simulink model "BiT_Template"  (R2025b)
settings: Solver=FixedStepAuto  StartTime=0.0  StopTime=40  FixedStep=0.005  RelTol=1e-3
StopFcn:
  | user_confirmed = true;
  | disp('Gestoppt?!')
  | 
  | % stop(t);
  | % delete(t);
  | 
  | %% Switch to Config Mode
  | %Tc3_AI.sysManager.ActivateConfiguration();
  | %
  | % Tc3_AI.SwitchToConfig('local')
  | %
  | % %save Solution
  | % Tc3_AI.SaveSolution();
  | %
  | % %% Close Aktive VS Instance
  | % Tc3_AI.closeVsInstance();
libraries: slpidlib x1
settings Model: SimulationMode=external  Creator=clemensm  LastModifiedBy=Felix
settings OptimizationCC: LocalBlockOutputs=off
settings RTWCC: SystemTargetFile=TwinCatGrt.tlc  GenCodeOnly=on  GenerateMakefile=off  TemplateMakefile=tcgrt_msbuild.tmf  TargetLang=C++  Description=TwinCAT GRT Target
settings STFCustomTargetCC: SystemTargetFile=TwinCatGrt.tlc  TargetLangStandard=C++11 (ISO)  CombineOutputUpdateFcns=on  CodeInterfacePackaging=Reusable function  CPPClassGenCompliant=on  GRTInterface=off  GenerateAllocFcn=on  TcCom_BlockDiagramExport=on  TcCom_Legacy_ModuleBuildInfoParam=on  TcCom_ExtModeRtWaitForStart=off  TcProject_LibraryCategories=$<VendorName>  TcCom_ExecutionSequence=UpdateBeforeOutputMapping  TcProject_UseTmxExtension=Auto  TcCom_OnlineChange=off  TcProject_ProjectDir=C:\TwinCAT\3.1\CustomConfig\Modules\Ctrl_only  TcCom_AllowDataAreaForSharedData=off  TcCom_TcComWrapperFb=off  TcProject_VendorIcon=$<TE140x:Icon>  TcProject_Copyright=Copyright $<VendorName> $<LocalDateTime:%Y>  TcProject_UseNativeBlockDiagramExport=off  TcProject_LowestCompatibleTcBuild=$<TwinCAT:Version:BUILD>  TcCom_BlockIoDataAccess=Internal DataArea  TcCom_ModuleIcon=$<TE140x:Icon>  TcPlcFb_ExtModeRtWaitForStart=off  TcPlcFb_ExtModeRtAllowExecutionCommands=off  TcCom_DataStoreReadOnly=off  TcProject_GenerateStructDutsWithDefaultValues=Auto  TcProject_InstallPlcLibrary=off  TcPlcFb_ExtModeRtAllowForParameterChange=off  TcPlcFb_InitExceptionHandling=CallerExceptions  TcCom_ExecutionInfoParam=on  TcCom_DWorkReadOnly=on  TcCom_CallerVerification=Default  TcProject_BuildWithWdk=inherit default  TcCom_BlockDiagramVariableAccess=AssignToParent  TcCom_TcComWrapperFbProperties=off  TcProject_UseIntrinsics=on  TcCom_InputCreateSymbols=on  TcProject_ForceRebuildForPublish=off  TcProject_CLanguageStandard=Default  TcCom_DWorkCreateSymbols=on  TcCom_OemLicenses=$<Project:OemLicenses>  TcCom_ExtendSignalResolution=on  TcProject_PublishTcOSARMv7M=off  TcProject_PreferToolArchitectureX64=on  TcCom_StepSizeAdaptation=RequireMatchingTaskCycleTime  TcPlcFb_Generate=off  TcCom_OnlineChangeRestoreDataAreas=off  TcProject_PreferIntOverLong=off  TcProject_CoderCppNamespace=coder  TcProject_Generate=on  TcCom_OutputReadOnly=on  TcProject_CreateUniqueEnumItemNames=off  TcCom_DataStoreCreateSymbols=on  TcProject_UseDescriptorCodeType=on  TcCom_TcComWrapperFbPropertyMonitoring=NoMonitoring  TcProject_UseStaticStlString=off  TcProject_Description=TwinCAT executable file, generated by TwinCAT $<ModuleGenerator:ProductId>  TcPlcFb_MonitorExecutionTime=off  TcCom_DWorkDataAccess=Internal DataArea  TcCom_InputInitValues=off  TcProject_UseCodeDescriptor=on  TcCom_GlobalParamDefaultSharing=Define  TcCom_BlockDiagramDebugInfoExport=on  TcProject_SignTwinCatCertName=MCI_2024_OEM.tccert  TcProject_StaticStlStringCapacity=Auto  TcCom_ContStateReadOnly=on  TcCom_UpdateExceptionHandling=CallerExceptions  TcProject_DrvFileVersion=$<VersionFromFile>  TcCom_ExtModeRtAllowForParameterChange=on  TcCom_VariableSymbolMapping=Identical  TcCom_BlockIoReadOnly=on  TcCom_ExecuteModelCode=on  TcCom_OutputDataAccess=Output Source DataArea  TcCom_BlockIoCreateSymbols=on  TcProject_GeneratePlcLibrary=off  TcProject_PublishTcOSARMv8A=off  TcProject_PublishTcOSx64=off  TcProject_DeployRestart=off  TcProject_ClassFactoryName=$<Project:Name>  TcProject_PublishConfiguration=Release  TcProject_IncrementVersion=Revision  TcProject_Versioning=Versioned  TcProject_BuildSystem=Auto  TcCom_ExtModeRtAllowExecutionCommands=on  TcProject_LibCatPath=$<Project:Dir>\$<Project:Name>.libcat.xml  TcCom_ParametersDataAccess=Internal DataArea  TcCom_ModuleCaller=CyclicTask  TcProject_TmxInstall=on  TcProject_PublishParallel=on  TcCom_ParametersInitValues=on  TcCom_AccessLockState=Auto  TcCom_InitExceptionHandling=CallerExceptions  TcCom_GroupDisplayName=$<GroupName>  TcCom_Generate=on  TcProject_PublishTcRTx86=on  TcProject_ProductName=$<ModuleGenerator:ProductId> $<ModuleGenerator:Version:MAJOR.MINOR>  TcCom_ExecutionInfoOutput=off  TcCom_GroupName=TE140x|Simulink Modules  TcProject_VersionSrc=$<LatestTMFile>  TcCom_ParametersCreateSymbols=on  TcCom_InputReadOnly=off  TcProject_PlcVarPrefixes=PVOID=p | BOOL=b | BOOL32=b | DATE=d | TIME_OF_DATE=td | TIME=t | LTIME=t | GUID=n  TcProject_Verbosity=Normal  TcProject_UseCodeInfoExporter=on  TcPlcFb_OemLicenses=$<Project:OemLicenses>  TcPlcFb_UpdateExceptionHandling=CallerExceptions  TcCom_StrictAccessLock=on  TcProject_Publish=on  TcCom_OriginalIoBlockNames=off  TcCom_ContStateDataAccess=Internal DataArea  TcCom_ResolveMaskedSubsystems=on  TcProject_MaxVisibleArrayElements=200U  TcCom_OutputCreateSymbols=on  TcProject_GenerateVsSolution=No  TcCom_DataStoreDataAccess=None  TcProject_PublishTcOSARMv7A=off  TcProject_CreateScopedEnums=Auto  TcCom_ParametersReadOnly=off  TcProject_SignWithTwinCatCertificate=inherit default  TcProject_PublishTcRTx64=on  TcProject_PublishPlatformtoolset=Auto  TcProject_EnableNewPlatforms=off  TcProject_DrvProductVersion=$<DrvFileVersion>  TcProject_PublishTcUMx86=off  TcProject_CppLanguageStandard=Default  TcCom_ContStateCreateSymbols=on  TcCom_InputDataAccess=Input Destination DataArea  TcCom_MonitorExecutionTime=off  TcProject_PublishTcUMx64=off  TcCom_GroupIcon=$<TE140x:Icon>  TcProject_DataExchangeModulesVersion=$<ModuleGenerator:DataExchange:Version>  TcProject_VendorName=TE140x Module Vendor  TcProject_UseDataExchangeModules=off
settings GRTTargetCC: ExtMode=on  ExtModeMexFile=TcExtModeClient  MultiInstanceErrorCode=None  TargetLangStandard=C++11 (ISO)  ParMdlRefBuildCompliant=off  CompOptLevelCompliant=off  MatFileLogging=off  CodeInterfacePackaging=Reusable function  GenerateAllocFcn=on  UseToolchainInfoCompliant=off

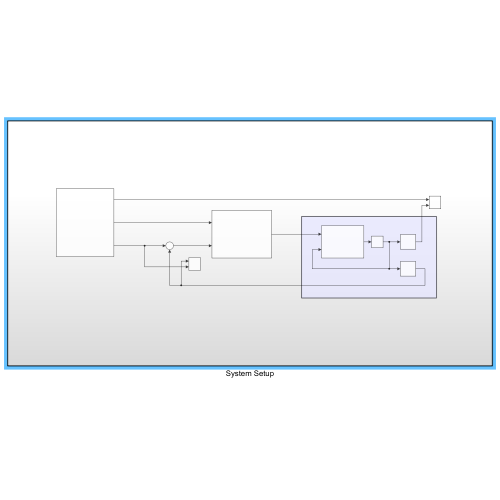
[thumbnail: Simulink's stored preview of the top-level diagram]
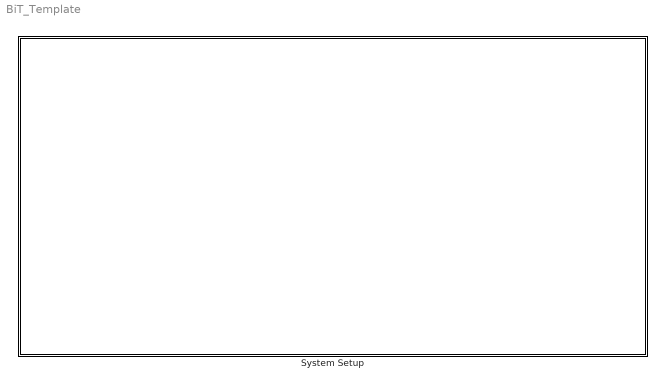
== system BiT_Template ==
  System Setup : Subsystem

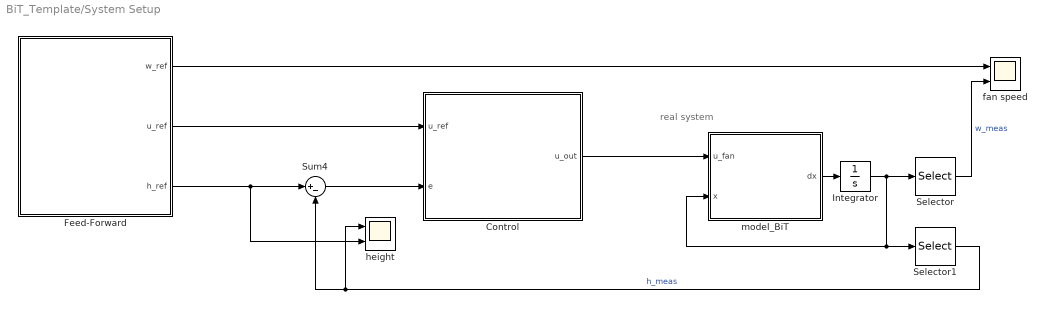
== system BiT_Template/System Setup ==
  note: real system
  Control : Subsystem
  Feed-Forward : Subsystem
  Integrator : Integrator
  Selector : Selector  InputPortWidth=3  IndexOptions=Index vector (dialog)  Indices=3  OutputSizes=1
  Selector1 : Selector  InputPortWidth=3  IndexOptions=Index vector (dialog)  Indices=1  OutputSizes=1
  Sum4 : Sum  Inputs=|+-
  fan speed : Scope  NumInputPorts=2
      settings: TimeSpan=60  ActiveDisplayYMinimum=4277  ActiveDisplayYMaximum=4777
  height : Scope  NumInputPorts=2
      settings: TimeSpan=60  ActiveDisplayYMinimum=-11.896668737884474  ActiveDisplayYMaximum=60.683450511895956  DataLoggingVariableName=ScopeData2
  model_BiT : MATLAB Function  TreatAsAtomicUnit=on
  wires:
  Selector1/1 -> height/1, Sum4/2  "h_meas"
  Selector/1 -> fan speed/2  "w_meas"
  model_BiT/1(dx) -> Integrator/1
  Integrator/1 -> Selector/1, Selector1/1, model_BiT/2(x)
  Feed-Forward/3(h_ref) -> height/2, Sum4/1
  Feed-Forward/1(w_ref) -> fan speed/1
  Feed-Forward/2(u_ref) -> Control/1(u_ref)
  Sum4/1 -> Control/2(e)
  Control/1(u_out) -> model_BiT/1(u_fan)

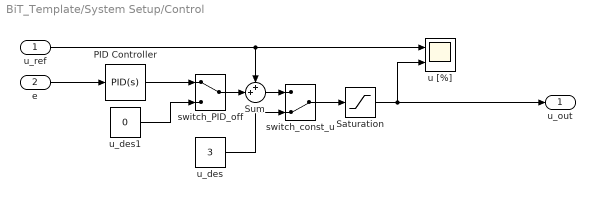
== system BiT_Template/System Setup/Control ==
  u_ref : Inport
  e : Inport  Port=2
  PID Controller : slpidlib/PID Controller  Controller=PID  Form=Parallel  TimeDomain=Continuous-time  UseExternalTs=off  SampleTime=-1  IntegratorMethod=Forward Euler  FilterMethod=Forward Euler  ControllerParametersSource=internal  P=1  I=1  UseKiTs=off  D=0  UseExternalDerivativeSource=off  N=100  UseFilter=on  TunerSelectOption=Transfer Function Based (PID Tuner App)  InitialConditionSource=internal  InitialConditionForIntegrator=0  InitialConditionForFilter=0  DifferentiatorICPrevScaledInput=0  ExternalReset=none  TrackingMode=off  Kt=1  LimitOutput=off  SatLimitsSource=internal  UpperSaturationLimit=inf  LowerSaturationLimit=-inf  LinearizeAsGain=on  AntiWindupMode=none  Kb=1  LimitIntegrator=off  UpperIntegratorSaturationLimit=inf  LowerIntegratorSaturationLimit=-inf  POutMin=[]  POutMax=[]  IOutMin=[]  IOutMax=[]  DOutMin=[]  DOutMax=[]  NOutMin=[]  NOutMax=[]  SumOutMin=[]  SumOutMax=[]  SaturationOutMin=[]  SaturationOutMax=[]  PParamMin=[]  PParamMax=[]  IParamMin=[]  IParamMax=[]  DParamMin=[]  DParamMax=[]  NParamMin=[]  NParamMax=[]  KbParamMin=[]  KbParamMax=[]  KtParamMin=[]  KtParamMax=[]  KbOutMin=[]  KbOutMax=[]  KtOutMin=[]  KtOutMax=[]  IntegratorOutMin=[]  IntegratorOutMax=[]  FilterOutMin=[]  FilterOutMax=[]  SumI1OutMin=[]  SumI1OutMax=[]  SumI2OutMin=[]  SumI2OutMax=[]  SumI3OutMin=[]  SumI3OutMax=[]  SumI4OutMin=[]  SumI4OutMax=[]  SumDOutMin=[]  SumDOutMax=[]  DifferentiatorOutMin=[]  DifferentiatorOutMax=[]  FilterDiffOutCoefMin=[]  FilterDiffOutCoefMax=[]  ReciprocalOutMin=[]  ReciprocalOutMax=[]  SumDenOutMin=[]  SumDenOutMax=[]  SumNumOutMin=[]  SumNumOutMax=[]  DivideOutMin=[]  DivideOutMax=[]  UdiffTsProdOutMin=[]  UdiffTsProdOutMax=[]  NTsProdOutMin=[]  NTsProdOutMax=[]  UintegralTsProdOutMin=[]  UintegralTsProdOutMax=[]  UngainTsProdOutMin=[]  UngainTsProdOutMax=[]  ClampingZeroOutDataTypeStr=Inherit: Inherit via back propagation  ClampingZeroOutMin=[]  ClampingZeroOutMax=[]  FilterDenConstantOutDataTypeStr=Inherit: Inherit via back propagation  FilterDenConstantOutMin=[]  FilterDenConstantOutMax=[]  PCopyOutDataTypeStr=Inherit: Inherit via back propagation  PCopyOutMin=[]  PCopyOutMax=[]  NCopyOutDataTypeStr=Inherit: Inherit via back propagation  NCopyOutMin=[]  NCopyOutMax=[]  IntegratorContinuousStateAttributes=''  IntegratorStateMustResolveToSignalObject=off  IntegratorRTWStateStorageClass=Auto  FilterContinuousStateAttributes=''  FilterStateMustResolveToSignalObject=off  FilterRTWStateStorageClass=Auto  ParallelPVariant=InternalParameters  IdealPVariant=Disabled  IVariant=InternalParameters  DVariant=InternalParameters  IntegratorVariant=Continuous  SatVariant=Disabled  AWVariant=Passthrough  PCopyVariant=Disabled  TRVariant=Disabled  FdbkBlocksVariant=Forward  IdealPFdbkVariant=Disabled  SatFdbkVariant=Disabled  DerivativeFilterVariant=ContFilter  NVariant=InternalParameters  NCopyVariant=Disabled  FilterICVariant=InternalICsFilter  IntegratorICVariant=InternalICs  ExternalResetVariant=Disabled  TRSumVariant=Passthrough  SumFdbkVariant=Disabled  SumVariant=Sum_PID  TsampFilterVariant=InternalTs  TsampNgainVariant=Passthrough  TsampIntegralVariant=Disabled_SignalSpec  ExternalSaturationOutDataTypeStr=Inherit: Same as second input  DerivativeSourceVariant=ErrorSignal  PreIntVariant=InternalPreInt
  Saturation : Saturate  UpperLimit=10  LowerLimit=0
  Sum : Sum  Inputs=++|
  switch_PID_off : ManualSwitch
  switch_const_u : ManualSwitch  CurrentSetting=0
  u [%] : Scope  NumInputPorts=2
      settings: TimeSpan=60  ActiveDisplayYMinimum=1.6341767510650569  ActiveDisplayYMaximum=6.6167058635554366
  u_des : Constant  Value=3
  u_des1 : Constant  Value=0
  u_out : Outport
  wires:
  u_des/1 -> switch_const_u/2
  Saturation/1 -> u_out/1, u [%]/2
  e/1 -> PID Controller/1
  switch_const_u/1 -> Saturation/1
  u_ref/1 -> u [%]/1, Sum/1
  Sum/1 -> switch_const_u/1
  PID Controller/1 -> switch_PID_off/1
  switch_PID_off/1 -> Sum/2
  u_des1/1 -> switch_PID_off/2

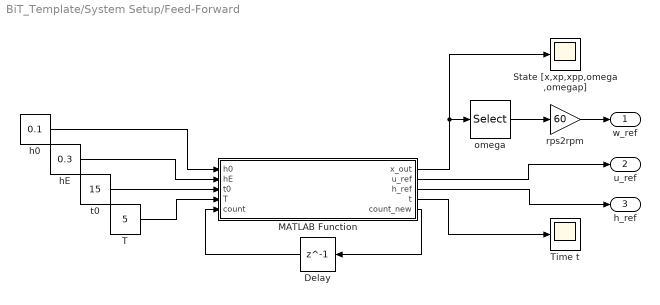
== system BiT_Template/System Setup/Feed-Forward ==
  Delay : Delay  DelayLength=1
  MATLAB Function : MATLAB Function  TreatAsAtomicUnit=on
  State [x,xp,xpp,omega,omegap] : Scope
      settings: TimeSpan=60  ActiveDisplayYMinimum=-34.55818  ActiveDisplayYMaximum=92.49741
  T : Constant  Value=5
  Time t : Scope
      settings: ActiveDisplayYMinimum=-17.36  ActiveDisplayYMaximum=-4.86
  h0 : Constant  Value=0.1
  hE : Constant  Value=0.3
  omega : Selector  InputPortWidth=5  IndexOptions=Index vector (dialog)  Indices=4  OutputSizes=1
  rps2rpm : Gain  Gain=60
  t0 : Constant  Value=15
  w_ref : Outport
  u_ref : Outport  Port=2
  h_ref : Outport  Port=3
  wires:
  h0/1 -> MATLAB Function/1(h0)
  omega/1 -> rps2rpm/1
  MATLAB Function/4(t) -> Time t/1
  T/1 -> MATLAB Function/4(T)
  t0/1 -> MATLAB Function/3(t0)
  Delay/1 -> MATLAB Function/5(count)
  MATLAB Function/5(count_new) -> Delay/1
  hE/1 -> MATLAB Function/2(hE)
  MATLAB Function/1(x_out) -> State [x,xp,xpp,omega,omegap]/1, omega/1
  MATLAB Function/2(u_ref) -> u_ref/1
  MATLAB Function/3(h_ref) -> h_ref/1
  rps2rpm/1 -> w_ref/1

== matlab function BiT_Template/System Setup/model_BiT ==
  data: u_fan input; dx output; x input
function dx = model_BiT(u_fan, x)
% Define constants as persistent or global variables if running
% outside of a script environment, or simply define them inside
% the function as they are constants.

    alpha1 = 0.0071;
    alpha2 = 0.2237;
    alpha3 = 9.8100;
    u0 = -1.1812;
    tau_w = 1.7217;
    k_w = 286.7462;
    
    % --- Explicitly initialize dx as a 3x1 column vector ---
    % Simulink needs to know the size of this output.
    dx = zeros(3,1); 
    
    % --- State Extraction ---
    x2 = x(2);          % x(2) = dz/dt
    x3 = x(3);          % x(3) = omega (fan speed)
    
    % --- Calculation of State Derivatives ---
    
    % 1. Height derivative (dx1/dt = dz/dt)
    dx(1) = x2; 

    % 2. Velocity derivative (dx2/dt = d^2z/dt^2) - Ball Dynamics
    dx(2) = (alpha1 * x3 - alpha2 * x2)^2 - alpha3;
    
    u_t = (u_fan/100)*5;

    % 3. Fan speed derivative (dx3/dt = d(omega)/dt) - Fan Dynamics
    dx(3) = (1 / tau_w) * (k_w * (u_t - u0) - x3);
    
end

== matlab function BiT_Template/System Setup/Feed-Forward/MATLAB Function ==
  data: x_out output; u_ref output; h0 input; hE input; t0 input; T input; h_ref output; t output; count input; count_new output
function [x_out,u_ref,h_ref,t,count_new] = feed_forward(h0,hE,t0,T,count)

count_new = count+1;
dT = 0.005;
t = count_new*dT-t0;

% Parameter



% Calculate Trajectory

xp_ref = 0;
xpp_ref = 0;
xppp_ref = 0;

if t<0
    x_ref = h0;
elseif t>T
    x_ref = hE;
else
    x_ref = h0; % Trajectory has to be implemented!
end

% Equations:
omega = 0; % equation for omega
omega_p = 0; % equation for omega
u = 0; % equation for omega

h_ref = x_ref;
u_ref = u; 
x_out = [x_ref,xp_ref,xpp_ref,omega,omega_p]';
end
